simulink model "mUnconnected"  (Simulink 7.1)
settings: Solver=ode3  StartTime=0.0  StopTime=10.0  FixedStep=0.1  RelTol=1e-3
settings Model: Creator=jcobleig  LastModifiedBy=jcobleig
settings OptimizationCC: InlineParams=on
settings DebuggingCC: StrictBusMsg=ErrorOnBusTreatedAsVector

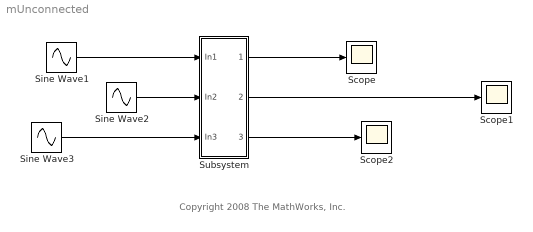
== system mUnconnected ==
  note: Copyright 2008 The MathWorks, Inc.
  Scope : Scope
  Scope1 : Scope
  Scope2 : Scope
      settings: SaveName=ScopeData2
  Sine Wave1 : Sin  Frequency=2  SampleTime=0.1
  Sine Wave2 : Sin  Frequency=2  SampleTime=0.1
  Sine Wave3 : Sin  Frequency=2  SampleTime=0.1
  Subsystem : Subsystem  TreatAsAtomicUnit=on
  wires:
  Subsystem/1(Out1) -> Scope/1
  Subsystem/2(Out2) -> Scope1/1
  Sine Wave1/1 -> Subsystem/1(In1)
  Subsystem/3(Out3) -> Scope2/1
  Sine Wave2/1 -> Subsystem/2(In2)
  Sine Wave3/1 -> Subsystem/3(In3)

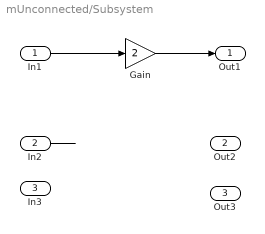
== system mUnconnected/Subsystem ==
  In1 : Inport
  In2 : Inport  Port=2
  In3 : Inport  Port=3
  Gain : Gain  Gain=2  ParameterDataType=sfix(16)  ParameterScaling=2^0  OutDataType=sfix(16)  OutScaling=2^0
  Out1 : Outport
  Out2 : Outport  Port=2
  Out3 : Outport  Port=3
  wires:
  In1/1 -> Gain/1
  Gain/1 -> Out1/1
  ? -> Out2/1
  In2/1 -> ?
